simulink model "ECE453Hw3"  (R2025a)
settings: Solver=FixedStepAuto  StartTime=0.0  StopTime=1  FixedStep=0.001  RelTol=1e-3
settings Model: Creator=cruisemac  LastModifiedBy=cruisemac
settings DataIOCC: SaveFinalState=on  SaveState=on  InspectSignalLogs=on  LoggingToFile=on

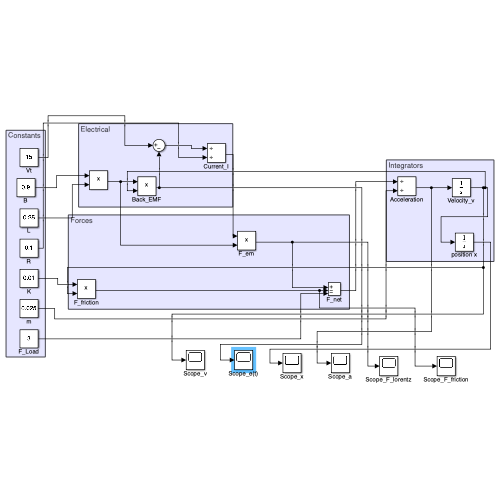
[thumbnail: Simulink's stored preview of the top-level diagram]
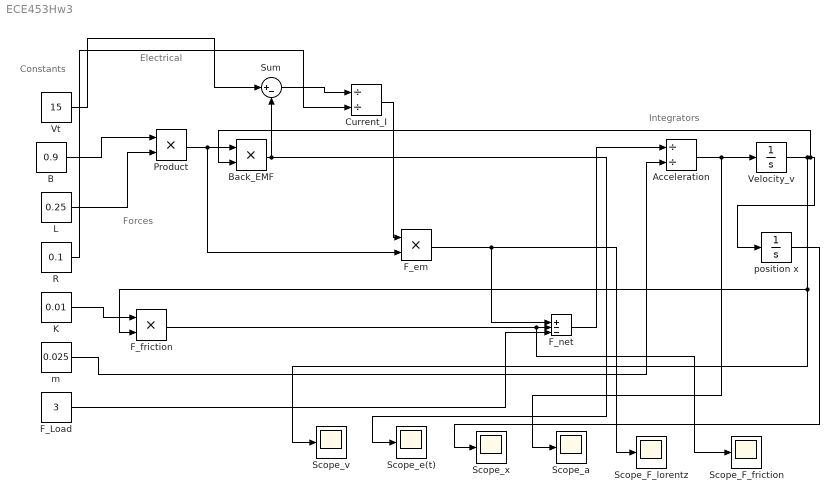
== system ECE453Hw3 ==
  note: Forces
  note: Integrators
  note: Electrical
  note: Constants
  Acceleration : Product  Inputs=//
  B : Constant  Value=0.9
  Back_EMF : Product
  Current_I : Product  Inputs=//
  F_Load : Constant  Value=3
  F_em : Product
  F_friction : Product
  F_net : Sum  Inputs=|+--
  K : Constant  Value=0.01
  L : Constant  Value=0.25
  Product : Product
  R : Constant  Value=0.1
  Scope_F_friction : Scope
      settings: ActiveDisplayYMinimum=-1  ActiveDisplayYMaximum=1  DataLoggingVariableName=ScopeData5
  Scope_F_lorentz : Scope
      settings: ActiveDisplayYMinimum=0.12038105953867066  ActiveDisplayYMaximum=0.15069050382026578  DataLoggingVariableName=ScopeData2
  Scope_a : Scope
      settings: ActiveDisplayYMinimum=-1  ActiveDisplayYMaximum=1  DataLoggingVariableName=ScopeData3
  Scope_e(t) : Scope
      settings: ActiveDisplayYMinimum=-3.6257785506861273  ActiveDisplayYMaximum=0.40286428340956959
  Scope_v : Scope
      settings: ActiveDisplayYMinimum=-26.180393808966237  ActiveDisplayYMaximum=0.81581374531033468
  Scope_x : Scope
      settings: ActiveDisplayYMinimum=-1  ActiveDisplayYMaximum=1  DataLoggingVariableName=ScopeData4
  Sum : Sum  Inputs=|+-
  Velocity_v : Integrator
  Vt : Constant  Value=15
  m : Constant  Value=0.025
  position x : Integrator
  wires:
  F_em/1 -> Scope_F_lorentz/1, F_net/1
  Back_EMF/1 -> Scope_e(t)/1, Sum/2
  Acceleration/1 -> Scope_a/1, Velocity_v/1
  position x/1 -> Scope_x/1
  Sum/1 -> Current_I/1
  B/1 -> Product/1
  R/1 -> Current_I/2
  L/1 -> Product/2
  Vt/1 -> Sum/1
  m/1 -> Acceleration/2
  F_net/1 -> Acceleration/1
  F_friction/1 -> Scope_F_friction/1, F_net/2
  Product/1 -> F_em/2, Back_EMF/1
  K/1 -> F_friction/1
  F_Load/1 -> F_net/3
  Velocity_v/1 -> F_friction/2, Scope_v/1, position x/1, Back_EMF/2
  Current_I/1 -> F_em/1
